simulink model "Sim2_test_var_load"  (R2018a)
settings: Solver=ode1  StartTime=0.0  StopTime=4  FixedStep=Time_Step  MaxStep=1e-4  RelTol=1e-3
undefined symbols (not defined in the file): Bxx_GenericVoltageSource, Lg, Rg, Source_Lib, Theta0, Time_Step, Ug, Un, V0, VSC01_id0
libraries: powerlib x29, simulink x8, Control_Lib x1
(part 2 of 2)

== system Sim2_test_var_load/VSC01/Control loops/ pu P//Q computation ==
  v_abc_pu : Inport  PortDimensions=3
  i_abc_pu : Inport  Port=2  PortDimensions=3
  Demux : Demux  Outputs=3
      settings: DisplayOption=none
  Mux : Mux  Inputs=3
  Product1 : Product  InputSameDT=on  SaturateOnIntegerOverflow=on  OutDataTypeStr=Inherit: Same as first input
  Product3 : Product  InputSameDT=on  SaturateOnIntegerOverflow=on  OutDataTypeStr=Inherit: Same as first input
  Sum : Sum  Inputs=+-  InputSameDT=on  SaturateOnIntegerOverflow=on  OutDataTypeStr=Inherit: Same as first input
  Sum1 : Sum  Inputs=1  InputSameDT=on  SaturateOnIntegerOverflow=on  OutDataTypeStr=Inherit: Same as first input
  Sum4 : Sum  Inputs=1  InputSameDT=on  SaturateOnIntegerOverflow=on  OutDataTypeStr=Inherit: Same as first input
  Sum5 : Sum  Inputs=+-  InputSameDT=on  SaturateOnIntegerOverflow=on  OutDataTypeStr=Inherit: Same as first input
  Sum6 : Sum  Inputs=+-  InputSameDT=on  SaturateOnIntegerOverflow=on  OutDataTypeStr=Inherit: Same as first input
  pu->V : Gain  Gain=1/sqrt(3)  SaturateOnIntegerOverflow=on  OutDataTypeStr=Inherit: Same as input  ParamDataTypeStr=Inherit: Same as input
  pu->V1 : Gain  Gain=1/3  SaturateOnIntegerOverflow=on  OutDataTypeStr=Inherit: Same as input  ParamDataTypeStr=Inherit: Same as input
  pu->V2 : Gain  Gain=1/3  SaturateOnIntegerOverflow=on  OutDataTypeStr=Inherit: Same as input  ParamDataTypeStr=Inherit: Same as input
  P : Outport  VectorParamsAs1DForOutWhenUnconnected=off
  Q : Outport  Port=2  VectorParamsAs1DForOutWhenUnconnected=off
  wires:
  pu->V2/1 -> Q/1
  pu->V1/1 -> P/1
  Sum1/1 -> pu->V/1
  Product3/1 -> Sum1/1
  Product1/1 -> Sum4/1
  v_abc_pu/1 -> Product1/1, Demux/1
  i_abc_pu/1 -> Product1/2, Product3/2
  Sum4/1 -> pu->V1/1
  Demux/1 -> Sum/1, Sum6/2
  Demux/2 -> Sum/2, Sum5/1
  Demux/3 -> Sum5/2, Sum6/1
  Sum/1 -> Mux/3
  Sum5/1 -> Mux/1
  Sum6/1 -> Mux/2
  Mux/1 -> Product3/1
  pu->V/1 -> pu->V2/1  "Q"

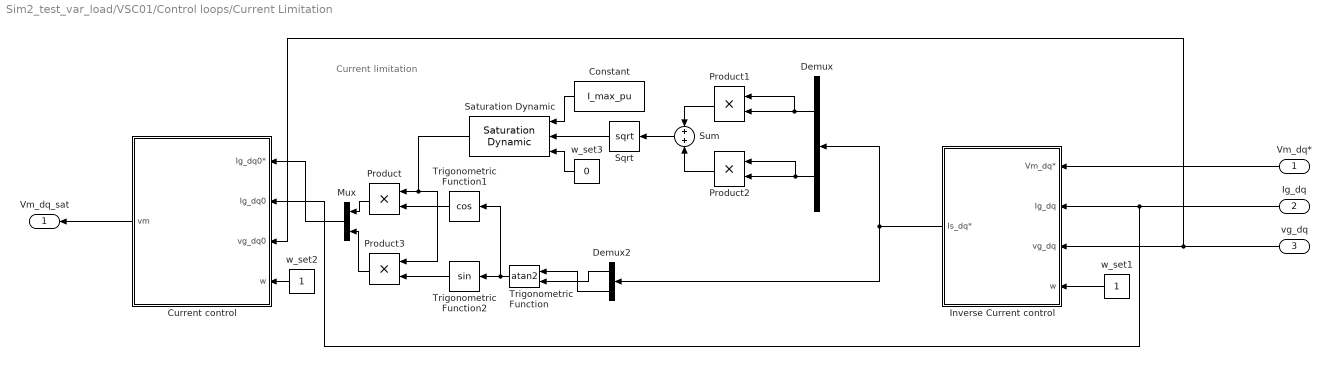
== system Sim2_test_var_load/VSC01/Control loops/Current Limitation ==
  note: Current limitation
  Vm_dq* : Inport
  Ig_dq : Inport  Port=2
  vg_dq : Inport  Port=3
  Constant : Constant  Value=I_max_pu
  Current control : Subsystem
  Demux : Demux  Outputs=2
  Demux2 : Demux  Outputs=2
  Inverse Current control : Subsystem
  Mux : Mux  Inputs=2
  Product{,1..3} (4 alike) : Product
  Saturation Dynamic : simulink/Discontinuities/Saturation Dynamic  OutMin=[]  OutMax=[]  OutDataTypeStr=Inherit: Same as second input  OutDataType=fixdt(1, 16)  OutScaling=2^-10  DoSatur=off
  Sqrt : Sqrt  SaturateOnIntegerOverflow=on
  Sum : Sum
  Trigonometric Function : Trigonometry  Operator=atan2  NumberOfIterations=5  OutputSignalType=real
  Trigonometric Function1 : Trigonometry  Operator=cos
  Trigonometric Function2 : Trigonometry
  w_set1 : Constant
  w_set2 : Constant
  w_set3 : Constant  Value=0
  Vm_dq_sat : Outport  VectorParamsAs1DForOutWhenUnconnected=off
  wires:
  w_set3/1 -> Saturation Dynamic/3
  Constant/1 -> Saturation Dynamic/1
  Mux/1 -> Current control/1(Ig_dq0*)
  Product/1 -> Mux/1
  Demux/1 -> Product1/1, Product1/2
  Demux/2 -> Product2/1, Product2/2
  Trigonometric Function2/1 -> Product3/2
  Product2/1 -> Sum/2
  Trigonometric Function1/1 -> Product/2
  Demux2/1 -> Trigonometric Function/2
  Trigonometric Function/1 -> Trigonometric Function2/1, Trigonometric Function1/1
  Saturation Dynamic/1 -> Product/1, Product3/1
  Product1/1 -> Sum/1
  Sqrt/1 -> Saturation Dynamic/2
  Demux2/2 -> Trigonometric Function/1
  Inverse Current control/1(Is_dq*) -> Demux2/1, Demux/1
  Sum/1 -> Sqrt/1
  Product3/1 -> Mux/2
  Ig_dq/1 -> Inverse Current control/2(Ig_dq), Current control/2(Ig_dq0)
  w_set1/1 -> Inverse Current control/4(w)
  w_set2/1 -> Current control/4(w)
  vg_dq/1 -> Current control/3(vg_dq0), Inverse Current control/3(vg_dq)
  Vm_dq*/1 -> Inverse Current control/1(Vm_dq*)
  Current control/1(vm) -> Vm_dq_sat/1

== system Sim2_test_var_load/VSC01/Control loops/PLL ==
  abc_pu : Inport
  Demux : Demux  Outputs=[1 1]
  Mux : Mux  Inputs=2
  PI PLL controller : Subsystem
  Terminator1 : Terminator
  Terminator2 : Terminator
  Trigonometric Function : Trigonometry  Operator=cos
  Trigonometric Function1 : Trigonometry
  abc2dq0_norm : Subsystem  AncestorBlock=Control_Lib/abc2dq0_norm  TreatAsAtomicUnit=on  mask{referenceAxisMode=Reference axis at 90 degrees behind phase_a, baseUpdateGain=1/sqrt(3)}
      mask prompts: referenceAxisMode "Chosse reference axis of the angular position"; baseUpdateGain "Gain to update base from abc to dq0 frames"
      mask init: same as Sim2_test_var_load/VSC01/Control loops/abc2dq0_norm
      mask TypeOptions referenceAxisMode: Reference axis on phase_a | Reference axis at 90 degrees behind phase_a
      mask DialogControl DescGroupVar Prompt: CONFIGURATION
      mask DialogControl Container3 Prompt: Reference axis
      mask DialogControl Container4 Prompt: Base definition
      mask DialogControl Control1 Prompt: Gain = 1.0 : No base update
      mask DialogControl Control1_copy Prompt: Gain = 1/sqrt(3) : 1pu RMS in abc frame = 1pu in dq0 frame
  Theta_rad : Outport  PortDimensions=1  VectorParamsAs1DForOutWhenUnconnected=off
  CosSinTheta : Outport  Port=2  PortDimensions=2  VectorParamsAs1DForOutWhenUnconnected=off
  w_pu : Outport  Port=3  PortDimensions=1  VectorParamsAs1DForOutWhenUnconnected=off
  vd : Outport  Port=4  PortDimensions=1  VectorParamsAs1DForOutWhenUnconnected=off
  wires:
  Demux/1 -> vd/1
  Demux/2 -> PI PLL controller/1(vq)
  PI PLL controller/1(w) -> w_pu/1
  abc2dq0_norm/2(dq) -> Demux/1
  PI PLL controller/2(Theta) -> Trigonometric Function1/1, Trigonometric Function/1, Theta_rad/1
  Trigonometric Function1/1 -> Mux/2
  Trigonometric Function/1 -> Mux/1
  Mux/1 -> abc2dq0_norm/2(CosSinTheta), CosSinTheta/1
  abc_pu/1 -> abc2dq0_norm/1(abc)
  abc2dq0_norm/3(ZeroSequence) -> Terminator1/1
  abc2dq0_norm/1(AlphaBeta) -> Terminator2/1

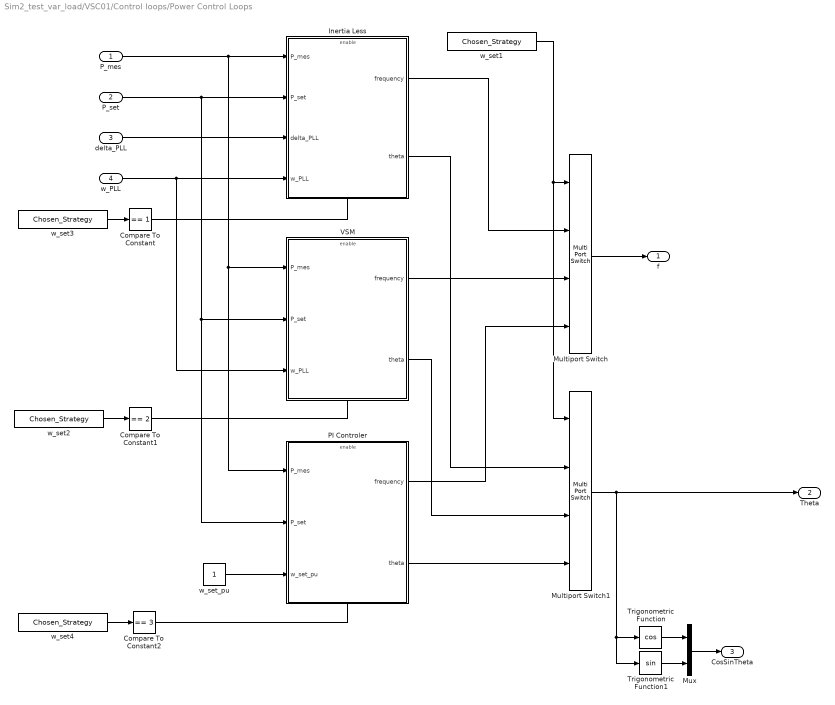
== system Sim2_test_var_load/VSC01/Control loops/Power Control Loops ==
  P_mes : Inport
  P_set : Inport  Port=2
  delta_PLL : Inport  Port=3
  w_PLL : Inport  Port=4
  Compare To Constant : simulink/Logic and Bit Operations/Compare To Constant  relop===  const=1  OutDataTypeStr=boolean
  Compare To Constant1 : simulink/Logic and Bit Operations/Compare To Constant  relop===  const=2  OutDataTypeStr=boolean
  Compare To Constant2 : simulink/Logic and Bit Operations/Compare To Constant  relop===  const=3  OutDataTypeStr=boolean
  Inertia Less : Subsystem
  Multiport Switch : MultiPortSwitch
  Multiport Switch1 : MultiPortSwitch
  Mux : Mux  Inputs=[1 1]
  PI Controler : Subsystem
  Trigonometric Function : Trigonometry  Operator=cos
  Trigonometric Function1 : Trigonometry
  VSM : Subsystem
  w_set{1..4} (4 alike) : Constant  Value=Chosen_Strategy
  w_set_pu : Constant
  f : Outport  PortDimensions=1  VectorParamsAs1DForOutWhenUnconnected=off
  Theta : Outport  Port=2  VectorParamsAs1DForOutWhenUnconnected=off
  CosSinTheta : Outport  Port=3  PortDimensions=2  VectorParamsAs1DForOutWhenUnconnected=off
  wires:
  Multiport Switch1/1 -> Trigonometric Function1/1, Trigonometric Function/1, Theta/1
  Trigonometric Function1/1 -> Mux/2
  Mux/1 -> CosSinTheta/1
  Trigonometric Function/1 -> Mux/1
  Compare To Constant2/1 -> PI Controler/Enable
  Compare To Constant1/1 -> VSM/Enable
  Compare To Constant/1 -> Inertia Less/Enable
  w_set4/1 -> Compare To Constant2/1
  w_set2/1 -> Compare To Constant1/1
  w_set3/1 -> Compare To Constant/1
  Inertia Less/1(frequency) -> Multiport Switch/2
  Multiport Switch/1 -> f/1
  Inertia Less/2(theta) -> Multiport Switch1/2
  VSM/2(theta) -> Multiport Switch1/3
  w_set1/1 -> Multiport Switch/1, Multiport Switch1/1
  VSM/1(frequency) -> Multiport Switch/3
  PI Controler/1(frequency) -> Multiport Switch/4
  PI Controler/2(theta) -> Multiport Switch1/4
  w_set_pu/1 -> PI Controler/3(w_set_pu)
  w_PLL/1 -> Inertia Less/4(w_PLL), VSM/3(w_PLL)
  delta_PLL/1 -> Inertia Less/3(delta_PLL)
  P_set/1 -> Inertia Less/2(P_set), VSM/2(P_set), PI Controler/2(P_set)
  P_mes/1 -> Inertia Less/1(P_mes), VSM/1(P_mes), PI Controler/1(P_mes)

== system Sim2_test_var_load/VSC01/Control loops/Transient Damping Resistance ==
  ig_dq : Inport
  Filter w_LF : Subsystem
      mask Display: disp('\omega_{LF} / (s + \omega_{LF})','texmode','on')
  Sum5 : Sum  Inputs=|+-
  nq1 : Gain  Gain=Rv
  "Delta_E_dq " : Outport  VectorParamsAs1DForOutWhenUnconnected=off
  wires:
  nq1/1 -> Filter w_LF/1(e), Sum5/2
  Filter w_LF/1(s) -> Sum5/1
  Sum5/1 -> "Delta_E_dq "/1
  ig_dq/1 -> nq1/1

== system Sim2_test_var_load/VSC01/Control loops/VI ==
  note: VI triggering and threshold computation
  note: VI
  i_VI_dq : Inport
  Demux1 : Demux  Outputs=2
      settings: DisplayOption=none
  Gain5 : Gain  Gain=DX_DR
  Gain6 : Gain  Gain=Kp_Rvi_pu
  Gain9 : Gain  Gain=DX_DR
  I_thresh : Constant  Value=I_thresh_pu
  Mux2 : Mux  Inputs=2
  Saturation : Saturate  UpperLimit=inf  LowerLimit=0
  Sum1 : Sum  Inputs=-+|
  Sum7 : Sum  Inputs=|+-
  Sum8 : Sum  Inputs=++|
  dq to phasor : Subsystem
  product{,1..3} (4 alike) : Product  InputSameDT=on  RndMeth=Zero  SaturateOnIntegerOverflow=on  OutDataTypeStr=Inherit: Same as first input
  I_rms : Outport  VectorParamsAs1DForOutWhenUnconnected=off
  Delta_E_dq : Outport  Port=2  VectorParamsAs1DForOutWhenUnconnected=off
  wires:
  Sum1/1 -> Saturation/1
  dq to phasor/1(rms) -> Sum1/2, I_rms/1  "I_rms"
  Saturation/1 -> Gain6/1
  I_thresh/1 -> Sum1/1
  Mux2/1 -> Delta_E_dq/1
  Gain6/1 -> product3/2, product/1, product1/2, product2/2
  product3/1 -> Gain5/1
  product/1 -> Gain9/1
  Demux1/1 -> product1/1, product/2  "igd"
  Demux1/2 -> product2/1, product3/1  "igq"
  product1/1 -> Sum7/1
  Gain5/1 -> Sum7/2
  Gain9/1 -> Sum8/1
  product2/1 -> Sum8/2
  Sum7/1 -> Mux2/1
  Sum8/1 -> Mux2/2
  i_VI_dq/1 -> dq to phasor/1(dq_mes), Demux1/1

== system Sim2_test_var_load/VSC01/Control loops/abc2dq0_norm ==
  abc : Inport
  CosSinTheta : Inport  Port=2
  Add : Sum
  Add1 : Sum  Inputs=-+
  Compare To Constant : simulink/Logic and Bit Operations/Compare To Constant  relop===  const=1  OutDataTypeStr=boolean
  Constant : Constant  Value=referenceAxisMode  OutDataTypeStr=uint16
  Demux : Demux  Outputs=2
  Demux1 : Demux  Outputs=3
  Gain : Gain  Gain=Concordia33  Multiplication=Matrix(K*u)
  Gain1 : Gain  Gain=baseUpdateGain
  Mux : Mux  Inputs=2
  Product{,1..3} (4 alike) : Product
  RotationInv90Deg : Subsystem  VariantControl=ROTATIONINV90DEG
  Switch : Switch  Criteria=u2 ~= 0
  AlphaBeta : Outport  VectorParamsAs1DForOutWhenUnconnected=off
  dq : Outport  Port=2  VectorParamsAs1DForOutWhenUnconnected=off
  ZeroSequence : Outport  Port=3  VectorParamsAs1DForOutWhenUnconnected=off
  wires:
  Gain1/1 -> Gain/1
  Compare To Constant/1 -> Switch/2
  Constant/1 -> Compare To Constant/1
  RotationInv90Deg/1(CosSinThetaOut) -> Switch/3
  CosSinTheta/1 -> RotationInv90Deg/1(CosSinThetaIn), Switch/1
  Switch/1 -> Demux/1
  Demux/1 -> Product/2, Product3/2
  Product3/1 -> Add1/2
  Product1/1 -> Add/2
  Demux/2 -> Product1/2, Product2/2
  Add1/1 -> Mux/2
  Gain/1 -> Demux1/1, AlphaBeta/1
  Demux1/2 -> Product3/1, Product1/1  "beta"
  Mux/1 -> dq/1
  Demux1/3 -> ZeroSequence/1  "zero"
  Add/1 -> Mux/1
  Demux1/1 -> Product2/1, Product/1  "alpha"
  Product/1 -> Add/1
  Product2/1 -> Add1/1
  abc/1 -> Gain1/1

== system Sim2_test_var_load/VSC01/Control loops/abc2dq0_norm1 ==
  abc : Inport
  CosSinTheta : Inport  Port=2
  Add : Sum
  Add1 : Sum  Inputs=-+
  Compare To Constant : simulink/Logic and Bit Operations/Compare To Constant  relop===  const=1  OutDataTypeStr=boolean
  Constant : Constant  Value=referenceAxisMode  OutDataTypeStr=uint16
  Demux : Demux  Outputs=2
  Demux1 : Demux  Outputs=3
  Gain : Gain  Gain=Concordia33  Multiplication=Matrix(K*u)
  Gain1 : Gain  Gain=baseUpdateGain
  Mux : Mux  Inputs=2
  Product{,1..3} (4 alike) : Product
  RotationInv90Deg : Subsystem  VariantControl=ROTATIONINV90DEG
  Switch : Switch  Criteria=u2 ~= 0
  AlphaBeta : Outport  VectorParamsAs1DForOutWhenUnconnected=off
  dq : Outport  Port=2  VectorParamsAs1DForOutWhenUnconnected=off
  ZeroSequence : Outport  Port=3  VectorParamsAs1DForOutWhenUnconnected=off
  wires:
  Gain1/1 -> Gain/1
  Compare To Constant/1 -> Switch/2
  Constant/1 -> Compare To Constant/1
  RotationInv90Deg/1(CosSinThetaOut) -> Switch/3
  CosSinTheta/1 -> RotationInv90Deg/1(CosSinThetaIn), Switch/1
  Switch/1 -> Demux/1
  Demux/1 -> Product/2, Product3/2
  Product3/1 -> Add1/2
  Product1/1 -> Add/2
  Demux/2 -> Product1/2, Product2/2
  Add1/1 -> Mux/2
  Gain/1 -> Demux1/1, AlphaBeta/1
  Demux1/2 -> Product3/1, Product1/1  "beta"
  Mux/1 -> dq/1
  Demux1/3 -> ZeroSequence/1  "zero"
  Add/1 -> Mux/1
  Demux1/1 -> Product2/1, Product/1  "alpha"
  Product/1 -> Add/1
  Product2/1 -> Add1/1
  abc/1 -> Gain1/1

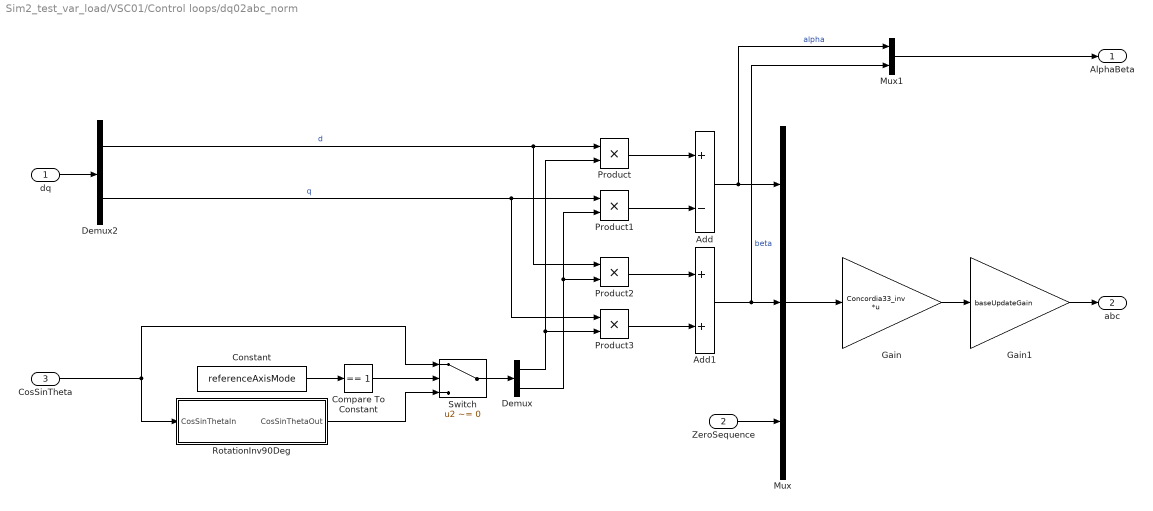
== system Sim2_test_var_load/VSC01/Control loops/dq02abc_norm ==
  dq : Inport
  ZeroSequence : Inport  Port=2
  CosSinTheta : Inport  Port=3
  Add : Sum  Inputs=+-
  Add1 : Sum
  Compare To Constant : simulink/Logic and Bit Operations/Compare To Constant  relop===  const=1  OutDataTypeStr=boolean
  Constant : Constant  Value=referenceAxisMode  OutDataTypeStr=uint16
  Demux : Demux  Outputs=2
  Demux2 : Demux  Outputs=2
  Gain : Gain  Gain=Concordia33_inv  Multiplication=Matrix(K*u)
  Gain1 : Gain  Gain=baseUpdateGain
  Mux : Mux  Inputs=3
  Mux1 : Mux  Inputs=2
  Product{,1..3} (4 alike) : Product
  RotationInv90Deg : Subsystem  VariantControl=ROTATIONINV90DEG
  Switch : Switch  Criteria=u2 ~= 0
  AlphaBeta : Outport  VectorParamsAs1DForOutWhenUnconnected=off
  abc : Outport  Port=2  VectorParamsAs1DForOutWhenUnconnected=off
  wires:
  Gain1/1 -> abc/1
  Constant/1 -> Compare To Constant/1
  RotationInv90Deg/1(CosSinThetaOut) -> Switch/3
  Demux/1 -> Product3/2, Product/2
  Mux/1 -> Gain/1
  Switch/1 -> Demux/1
  Demux/2 -> Product2/2, Product1/2
  Mux1/1 -> AlphaBeta/1
  Product/1 -> Add/1
  Demux2/2 -> Product1/1, Product3/1  "q"
  Add1/1 -> Mux/2, Mux1/2  "beta"
  Product1/1 -> Add/2
  Compare To Constant/1 -> Switch/2
  Product2/1 -> Add1/1
  Product3/1 -> Add1/2
  CosSinTheta/1 -> Switch/1, RotationInv90Deg/1(CosSinThetaIn)
  dq/1 -> Demux2/1
  ZeroSequence/1 -> Mux/3
  Demux2/1 -> Product/1, Product2/1  "d"
  Add/1 -> Mux/1, Mux1/1  "alpha"
  Gain/1 -> Gain1/1

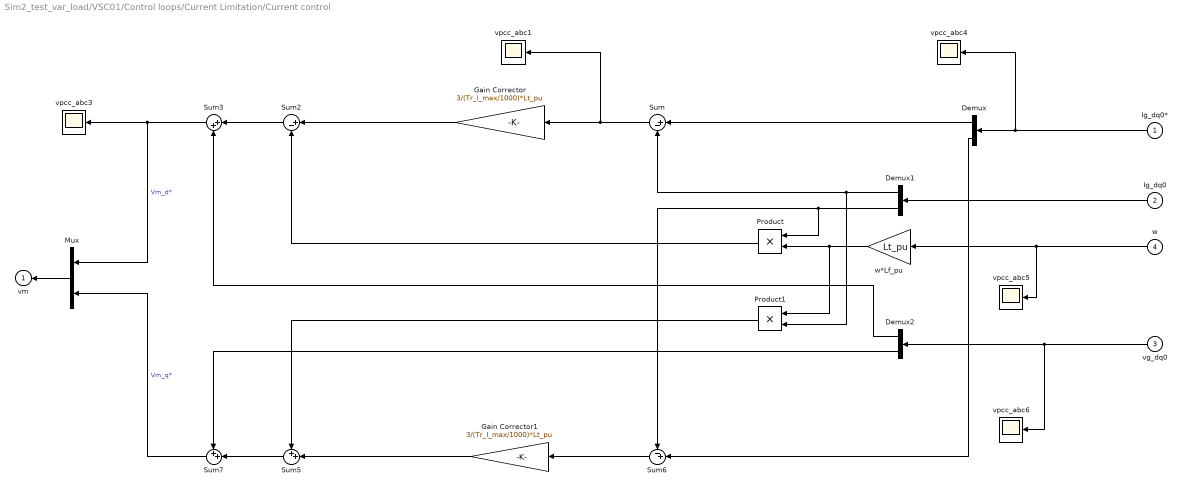
== system Sim2_test_var_load/VSC01/Control loops/Current Limitation/Current control ==
  Ig_dq0* : Inport
  Ig_dq0 : Inport  Port=2
  vg_dq0 : Inport  Port=3
  w : Inport  Port=4
  Demux : Demux  Outputs=2
  Demux1 : Demux  Outputs=2
  Demux2 : Demux  Outputs=2
  Gain Corrector : Gain  Gain=3/(Tr_I_max/1000)*Lt_pu
  Gain Corrector1 : Gain  Gain=3/(Tr_I_max/1000)*Lt_pu
  Mux : Mux  Inputs=2
  Product : Product  RndMeth=Zero
  Product1 : Product  RndMeth=Zero
  Sum : Sum  Inputs=|+-
  Sum2 : Sum  Inputs=|+-
  Sum3 : Sum  Inputs=|++
  Sum5 : Sum  Inputs=++|
  Sum6 : Sum  Inputs=-+|
  Sum7 : Sum  Inputs=++|
  vpcc_abc{1,3..6} (5 alike) : Scope
  w*Lf_pu : Gain  Gain=Lt_pu
  vm : Outport  InitialOutput=0  VectorParamsAs1DForOutWhenUnconnected=off
  wires:
  Demux2/2 -> Sum7/1
  Demux2/1 -> Sum3/2
  w/1 -> vpcc_abc5/1, w*Lf_pu/1
  Sum/1 -> vpcc_abc1/1, Gain Corrector/1
  Sum7/1 -> Mux/2  "Vm_q*"
  Sum3/1 -> Mux/1, vpcc_abc3/1  "Vm_d*"
  Sum5/1 -> Sum7/2
  Product1/1 -> Sum5/1
  Gain Corrector1/1 -> Sum5/2
  Demux/2 -> Sum6/2
  Sum2/1 -> Sum3/1
  Product/1 -> Sum2/2
  Demux1/2 -> Sum6/1, Product/1
  w*Lf_pu/1 -> Product/2, Product1/1
  Gain Corrector/1 -> Sum2/1
  Demux1/1 -> Sum/2, Product1/2
  Demux/1 -> Sum/1
  Ig_dq0/1 -> Demux1/1
  vg_dq0/1 -> Demux2/1, vpcc_abc6/1
  Sum6/1 -> Gain Corrector1/1
  Ig_dq0*/1 -> vpcc_abc4/1, Demux/1
  Mux/1 -> vm/1

== system Sim2_test_var_load/VSC01/Control loops/Current Limitation/Inverse Current control ==
  Vm_dq* : Inport
  Ig_dq : Inport  Port=2
  vg_dq : Inport  Port=3
  w : Inport  Port=4
  Demux : Demux  Outputs=2
  Demux1 : Demux  Outputs=2
  Demux2 : Demux  Outputs=2
  Gain Corrector2 : Gain  Gain=1/(3/(Tr_I_max/1000)*Lt_pu)
  Gain Corrector3 : Gain  Gain=1/(3/(Tr_I_max/1000)*Lt_pu)
  Mux : Mux  Inputs=2
  Product : Product  RndMeth=Zero
  Product1 : Product  RndMeth=Zero
  Sum : Sum  Inputs=|+-
  Sum2 : Sum  Inputs=|++
  Sum3 : Sum  Inputs=|++
  Sum5 : Sum  Inputs=-+|
  Sum6 : Sum  Inputs=-+|
  Sum7 : Sum  Inputs=++|
  w*Lf_pu : Gain  Gain=Lt_pu
  Is_dq* : Outport  InitialOutput=0  VectorParamsAs1DForOutWhenUnconnected=off
  wires:
  vg_dq/1 -> Demux2/1
  Ig_dq/1 -> Demux1/1
  Vm_dq*/1 -> Demux/1
  Demux/1 -> Sum/1
  Demux1/1 -> Sum3/2, Product1/2
  Sum/1 -> Sum2/1
  w*Lf_pu/1 -> Product1/1, Product/2
  Product/1 -> Sum2/2
  Sum2/1 -> Gain Corrector3/1
  Mux/1 -> Is_dq*/1
  Demux/2 -> Sum6/2
  Sum6/1 -> Sum5/2
  Sum5/1 -> Gain Corrector2/1
  Sum3/1 -> Mux/1  "is_d*"
  Sum7/1 -> Mux/2  "is_q*"
  w/1 -> w*Lf_pu/1
  Demux1/2 -> Sum7/1, Product/1
  Gain Corrector3/1 -> Sum3/1
  Demux2/1 -> Sum/2
  Demux2/2 -> Sum6/1
  Product1/1 -> Sum5/1
  Gain Corrector2/1 -> Sum7/2

== system Sim2_test_var_load/VSC01/Control loops/PLL/PI PLL controller ==
  vq : Inport
  0 - Vd1 : Gain  Gain=Kp_PLL  SaturateOnIntegerOverflow=on  OutDataTypeStr=Inherit: Same as input  ParamDataTypeStr=Inherit: Same as input
  0 - Vd2 : Gain  Gain=Ki_PLL  SaturateOnIntegerOverflow=on  OutDataTypeStr=Inherit: Same as input  ParamDataTypeStr=Inherit: Same as input
  Integrator : Integrator
  Integrator1 : Integrator  InitialCondition=Theta0*pi/180
  Sum : Sum  SaturateOnIntegerOverflow=on
  Sum1 : Sum  SaturateOnIntegerOverflow=on
  w_PLL_pu : Gain  Gain=wb  SaturateOnIntegerOverflow=on  OutDataTypeStr=Inherit: Same as input  ParamDataTypeStr=Inherit: Same as input
  w_set : Constant
  w : Outport  VectorParamsAs1DForOutWhenUnconnected=off
  Theta : Outport  Port=2  VectorParamsAs1DForOutWhenUnconnected=off
  wires:
  Integrator1/1 -> Theta/1
  0 - Vd2/1 -> Integrator/1
  w_set/1 -> Sum1/1
  w_PLL_pu/1 -> Integrator1/1
  Integrator/1 -> Sum/2
  Sum/1 -> Sum1/2
  0 - Vd1/1 -> Sum/1
  vq/1 -> 0 - Vd2/1, 0 - Vd1/1
  Sum1/1 -> w/1, w_PLL_pu/1

== system Sim2_test_var_load/VSC01/Control loops/PLL/abc2dq0_norm ==
  abc : Inport
  CosSinTheta : Inport  Port=2
  Add : Sum
  Add1 : Sum  Inputs=-+
  Compare To Constant : simulink/Logic and Bit Operations/Compare To Constant  relop===  const=1  OutDataTypeStr=boolean
  Constant : Constant  Value=referenceAxisMode  OutDataTypeStr=uint16
  Demux : Demux  Outputs=2
  Demux1 : Demux  Outputs=3
  Gain : Gain  Gain=Concordia33  Multiplication=Matrix(K*u)
  Gain1 : Gain  Gain=baseUpdateGain
  Mux : Mux  Inputs=2
  Product{,1..3} (4 alike) : Product
  RotationInv90Deg : Subsystem  VariantControl=ROTATIONINV90DEG
  Switch : Switch  Criteria=u2 ~= 0
  AlphaBeta : Outport  VectorParamsAs1DForOutWhenUnconnected=off
  dq : Outport  Port=2  VectorParamsAs1DForOutWhenUnconnected=off
  ZeroSequence : Outport  Port=3  VectorParamsAs1DForOutWhenUnconnected=off
  wires:
  Gain1/1 -> Gain/1
  Compare To Constant/1 -> Switch/2
  Constant/1 -> Compare To Constant/1
  RotationInv90Deg/1(CosSinThetaOut) -> Switch/3
  CosSinTheta/1 -> RotationInv90Deg/1(CosSinThetaIn), Switch/1
  Switch/1 -> Demux/1
  Demux/1 -> Product/2, Product3/2
  Product3/1 -> Add1/2
  Product1/1 -> Add/2
  Demux/2 -> Product1/2, Product2/2
  Add1/1 -> Mux/2
  Gain/1 -> Demux1/1, AlphaBeta/1
  Demux1/2 -> Product3/1, Product1/1  "beta"
  Mux/1 -> dq/1
  Demux1/3 -> ZeroSequence/1  "zero"
  Add/1 -> Mux/1
  Demux1/1 -> Product2/1, Product/1  "alpha"
  Product/1 -> Add/1
  Product2/1 -> Add1/1
  abc/1 -> Gain1/1

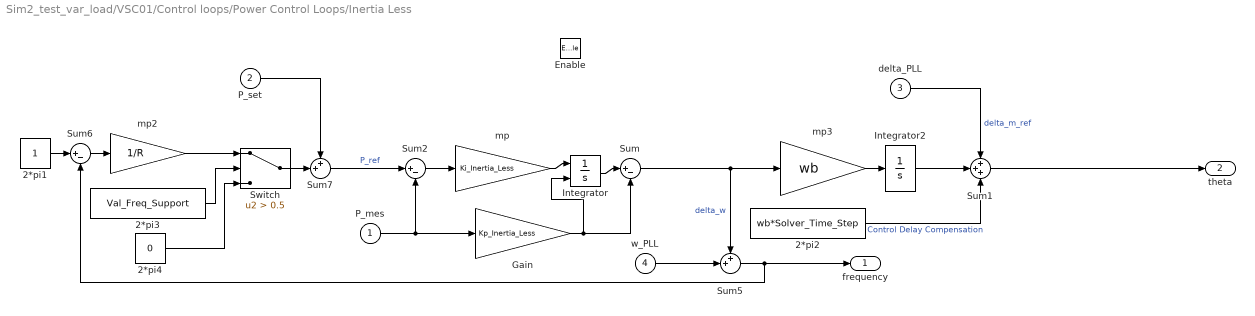
== system Sim2_test_var_load/VSC01/Control loops/Power Control Loops/Inertia Less ==
  P_mes : Inport
  P_set : Inport  Port=2
  delta_PLL : Inport  Port=3
  w_PLL : Inport  Port=4
  Enable : EnablePort
  2*pi1 : Constant
  2*pi2 : Constant  Value=wb*Solver_Time_Step
  2*pi3 : Constant  Value=Val_Freq_Support
  2*pi4 : Constant  Value=0
  Gain : Gain  Gain=Kp_Inertia_Less
  Integrator : Integrator  InitialConditionSource=external
  Integrator2 : Integrator  InitialCondition=(Theta_vsc0)*pi/180-Theta0*pi/180
  Sum : Sum  Inputs=|+-
  Sum1 : Sum  Inputs=+++
  Sum2 : Sum  Inputs=|+-
  Sum5 : Sum  Inputs=++|
  Sum6 : Sum  Inputs=|+-
  Sum7 : Sum  Inputs=++|
  Switch : Switch  Criteria=u2 > Threshold  Threshold=0.5
  mp : Gain  Gain=Ki_Inertia_Less
  mp2 : Gain  Gain=1/R
  mp3 : Gain  Gain=wb
  frequency : Outport  VectorParamsAs1DForOutWhenUnconnected=off
  theta : Outport  Port=2  VectorParamsAs1DForOutWhenUnconnected=off
  wires:
  Gain/1 -> Sum/2, Integrator/2
  Integrator/1 -> Sum/1
  2*pi4/1 -> Switch/3
  2*pi3/1 -> Switch/2
  mp2/1 -> Switch/1
  Integrator2/1 -> Sum1/2
  2*pi2/1 -> Sum1/3  "Control Delay Compensation"
  Sum5/1 -> Sum6/2, frequency/1
  w_PLL/1 -> Sum5/2
  delta_PLL/1 -> Sum1/1  "delta_m_ref"
  mp/1 -> Integrator/1
  mp3/1 -> Integrator2/1
  Sum/1 -> Sum5/1, mp3/1  "delta_w"
  Sum1/1 -> theta/1
  Switch/1 -> Sum7/2
  P_mes/1 -> Sum2/2, Gain/1
  Sum7/1 -> Sum2/1  "P_ref"
  P_set/1 -> Sum7/1
  Sum6/1 -> mp2/1
  2*pi1/1 -> Sum6/1
  Sum2/1 -> mp/1

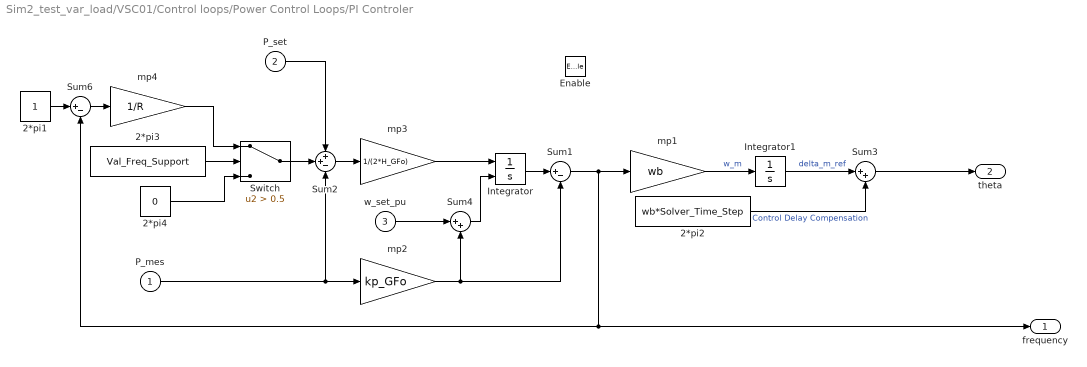
== system Sim2_test_var_load/VSC01/Control loops/Power Control Loops/PI Controler ==
  P_mes : Inport
  P_set : Inport  Port=2
  w_set_pu : Inport  Port=3
  Enable : EnablePort
  2*pi1 : Constant
  2*pi2 : Constant  Value=wb*Solver_Time_Step
  2*pi3 : Constant  Value=Val_Freq_Support
  2*pi4 : Constant  Value=0
  Integrator : Integrator  InitialConditionSource=external
  Integrator1 : Integrator  InitialCondition=(Theta_vsc0)*pi/180
  Sum1 : Sum  Inputs=|+-
  Sum2 : Sum  Inputs=++-
  Sum3 : Sum  Inputs=|++
  Sum4 : Sum  Inputs=|++
  Sum6 : Sum  Inputs=|+-
  Switch : Switch  Criteria=u2 > Threshold  Threshold=0.5
  mp1 : Gain  Gain=wb
  mp2 : Gain  Gain=kp_GFo
  mp3 : Gain  Gain=1/(2*H_GFo)
  mp4 : Gain  Gain=1/R
  frequency : Outport  VectorParamsAs1DForOutWhenUnconnected=off
  theta : Outport  Port=2  VectorParamsAs1DForOutWhenUnconnected=off
  wires:
  Switch/1 -> Sum2/2
  2*pi4/1 -> Switch/3
  Sum6/1 -> mp4/1
  2*pi3/1 -> Switch/2
  2*pi1/1 -> Sum6/1
  mp4/1 -> Switch/1
  Sum4/1 -> Integrator/2
  mp3/1 -> Integrator/1
  mp2/1 -> Sum4/2, Sum1/2
  P_mes/1 -> mp2/1, Sum2/3
  2*pi2/1 -> Sum3/2  "Control Delay Compensation"
  mp1/1 -> Integrator1/1  "w_m"
  Sum1/1 -> Sum6/2, frequency/1, mp1/1
  Integrator/1 -> Sum1/1
  P_set/1 -> Sum2/1
  w_set_pu/1 -> Sum4/1
  Integrator1/1 -> Sum3/1  "delta_m_ref"
  Sum2/1 -> mp3/1
  Sum3/1 -> theta/1

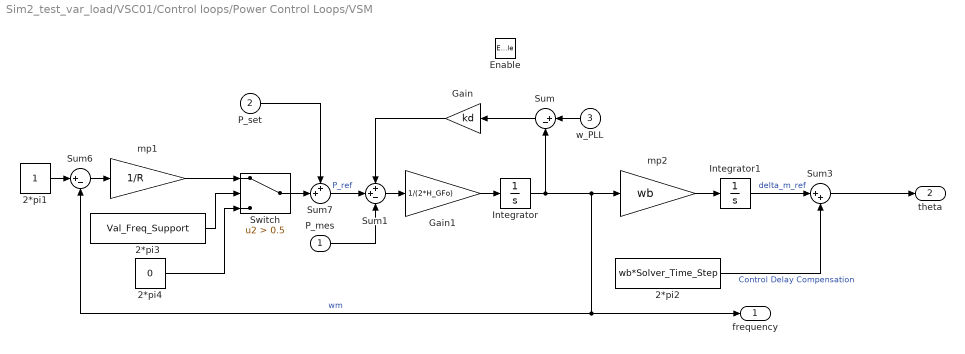
== system Sim2_test_var_load/VSC01/Control loops/Power Control Loops/VSM ==
  P_mes : Inport
  P_set : Inport  Port=2
  w_PLL : Inport  Port=3
  Enable : EnablePort
  2*pi1 : Constant
  2*pi2 : Constant  Value=wb*Solver_Time_Step
  2*pi3 : Constant  Value=Val_Freq_Support
  2*pi4 : Constant  Value=0
  Gain : Gain  Gain=kd
  Gain1 : Gain  Gain=1/(2*H_GFo)
  Integrator : Integrator  InitialCondition=1
  Integrator1 : Integrator  InitialCondition=Theta_vsc0*pi/180
  Sum : Sum  Inputs=|+-
  Sum1 : Sum  Inputs=++-
  Sum3 : Sum  Inputs=|++
  Sum6 : Sum  Inputs=|+-
  Sum7 : Sum  Inputs=++|
  Switch : Switch  Criteria=u2 > Threshold  Threshold=0.5
  mp1 : Gain  Gain=1/R
  mp2 : Gain  Gain=wb
  frequency : Outport  VectorParamsAs1DForOutWhenUnconnected=off
  theta : Outport  Port=2  VectorParamsAs1DForOutWhenUnconnected=off
  wires:
  Gain1/1 -> Integrator/1
  Sum7/1 -> Sum1/2  "P_ref"
  Sum1/1 -> Gain1/1
  Gain/1 -> Sum1/1
  Sum/1 -> Gain/1
  w_PLL/1 -> Sum/1
  2*pi4/1 -> Switch/3
  2*pi3/1 -> Switch/2
  mp1/1 -> Switch/1
  2*pi1/1 -> Sum6/1
  Sum6/1 -> mp1/1
  P_set/1 -> Sum7/1
  Switch/1 -> Sum7/2
  2*pi2/1 -> Sum3/2  "Control Delay Compensation"
  mp2/1 -> Integrator1/1
  P_mes/1 -> Sum1/3
  Integrator/1 -> Sum6/2, frequency/1, mp2/1, Sum/2  "wm"
  Integrator1/1 -> Sum3/1  "delta_m_ref"
  Sum3/1 -> theta/1

== system Sim2_test_var_load/VSC01/Control loops/Transient Damping Resistance/Filter w_LF ==
  e : Inport
  1/T_LP : Gain  Gain=W_TVR  SaturateOnIntegerOverflow=on  OutDataTypeStr=Inherit: Same as input  ParamDataTypeStr=Inherit: Same as input
  Integrator : Integrator  InitialConditionSource=external  InitialCondition=[VSC01_id0*0.04]
  Sum1 : Sum  Inputs=|+-  InputSameDT=on  SaturateOnIntegerOverflow=on  OutDataTypeStr=Inherit: Same as first input
  s : Outport  VectorParamsAs1DForOutWhenUnconnected=off
  wires:
  e/1 -> Sum1/1, Integrator/2
  Integrator/1 -> s/1, Sum1/2
  1/T_LP/1 -> Integrator/1
  Sum1/1 -> 1/T_LP/1

== system Sim2_test_var_load/VSC01/Control loops/VI/dq to phasor ==
  dq_mes : Inport
  Demux : Demux  Outputs=2
      settings: DisplayOption=none
  Sqrt : Sqrt  SaturateOnIntegerOverflow=on
  Sum4 : Sum  Inputs=|++  InputSameDT=on  SaturateOnIntegerOverflow=on  OutDataTypeStr=Inherit: Same as first input
  Vrdird : Product  InputSameDT=on  RndMeth=Zero  SaturateOnIntegerOverflow=on  OutDataTypeStr=Inherit: Same as first input
  Vrqirq : Product  InputSameDT=on  RndMeth=Zero  SaturateOnIntegerOverflow=on  OutDataTypeStr=Inherit: Same as first input
  rms : Outport  VectorParamsAs1DForOutWhenUnconnected=off
  wires:
  Sum4/1 -> Sqrt/1
  Vrqirq/1 -> Sum4/2
  Vrdird/1 -> Sum4/1
  Demux/2 -> Vrqirq/2, Vrqirq/1
  Demux/1 -> Vrdird/2, Vrdird/1
  dq_mes/1 -> Demux/1
  Sqrt/1 -> rms/1

== system Sim2_test_var_load/VSC01/Control loops/abc2dq0_norm/RotationInv90Deg ==
  CosSinThetaIn : Inport
  Demux : Demux  Outputs=2
  Gain1 : Gain  Gain=-1
  Mux : Mux  Inputs=2
  CosSinThetaOut : Outport  VectorParamsAs1DForOutWhenUnconnected=off
  wires:
  Gain1/1 -> Mux/2
  Demux/2 -> Mux/1
  Demux/1 -> Gain1/1
  CosSinThetaIn/1 -> Demux/1
  Mux/1 -> CosSinThetaOut/1

== system Sim2_test_var_load/VSC01/Control loops/abc2dq0_norm1/RotationInv90Deg ==
  CosSinThetaIn : Inport
  Demux : Demux  Outputs=2
  Gain1 : Gain  Gain=-1
  Mux : Mux  Inputs=2
  CosSinThetaOut : Outport  VectorParamsAs1DForOutWhenUnconnected=off
  wires:
  Gain1/1 -> Mux/2
  Demux/2 -> Mux/1
  Demux/1 -> Gain1/1
  CosSinThetaIn/1 -> Demux/1
  Mux/1 -> CosSinThetaOut/1

== system Sim2_test_var_load/VSC01/Control loops/dq02abc_norm/RotationInv90Deg ==
  CosSinThetaIn : Inport
  Demux1 : Demux  Outputs=2
  Gain1 : Gain  Gain=-1
  Mux1 : Mux  Inputs=2
  CosSinThetaOut : Outport  VectorParamsAs1DForOutWhenUnconnected=off
  wires:
  Demux1/2 -> Mux1/1
  CosSinThetaIn/1 -> Demux1/1
  Mux1/1 -> CosSinThetaOut/1
  Demux1/1 -> Gain1/1
  Gain1/1 -> Mux1/2

== system Sim2_test_var_load/VSC01/Control loops/PLL/abc2dq0_norm/RotationInv90Deg ==
  CosSinThetaIn : Inport
  Demux : Demux  Outputs=2
  Gain1 : Gain  Gain=-1
  Mux : Mux  Inputs=2
  CosSinThetaOut : Outport  VectorParamsAs1DForOutWhenUnconnected=off
  wires:
  Gain1/1 -> Mux/2
  Demux/2 -> Mux/1
  Demux/1 -> Gain1/1
  CosSinThetaIn/1 -> Demux/1
  Mux/1 -> CosSinThetaOut/1
